simulink model "abs_SLX_CS9"  (R2020a)
settings: Solver=ode45  StartTime=0  StopTime=10  FixedStep=0.001  RelTol=1e-3  AbsTol=1e-6
libraries: Solver_SF x1
settings Model: ExtModeTrigMode=oneshot  ExtModeArmWhenConnect=off  Creator=jhu  LastModifiedBy=S288668
settings SolverCC: AutoScaleAbsTol=off
settings DataIOCC: SaveFormat=Array  SignalLoggingSaveFormat=ModelDataLogs  ReturnWorkspaceOutputs=off  SignalLoggingName=sigsOut
settings OptimizationCC: BlockReduction=off  BooleanDataType=off  ExpressionDepthLimit=2147483647  LifeSpan=inf
settings DebuggingCC: SaveWithParameterizedLinksMsg=none  UnderspecifiedInitializationDetection=Classic  MergeDetectMultiDrivingBlocksExec=none  SignalResolutionControl=TryResolveAllWithWarning  MultiTaskDSMMsg=warning  MultiTaskCondExecSysMsg=none  FcnCallInpInsideContextMsg=warning  StateNameClashWarn=warning  SFUnexpectedBacktrackingDiag=warning  SFNoUnconditionalDefaultTransitionDiag=warning  SFExecutionAtInitializationDiag=none  ArithmeticOperatorsInVariantConditions=warning
settings HardwareCC: ProdBitPerPointer=32  ProdBitPerSizeT=32  ProdBitPerPtrDiffT=32  ProdLargestAtomicFloat=None  ProdIntDivRoundTo=Undefined  ProdEndianess=Unspecified  ProdWordSize=32  ProdHWDeviceType=32-bit Generic  TargetUnknown=on
settings ModelReferenceCC: PropagateSignalLabelsOutOfModel=off
settings SFSimCC: SimUseLocalCustomCode=off  CustomCodeUndefinedFunction=UseInterfaceOnly
settings RTWCC: TemplateMakefile=grt_vc.tmf  RTWUseLocalCustomCode=off
settings CodeAppCC: StateflowObjectComments=on
settings GRTTargetCC: TargetFcnLib=ansi_tfl_tmw.mat  TargetLangStandard=C89/C90 (ANSI)  CombineOutputUpdateFcns=off  GRTInterface=on
settings ConfigComp: CovMetricSettings=dw  CovHtmlReporting=on  CovSaveCumulativeToWorkspaceVar=on  CovSaveSingleToWorkspaceVar=on  CovExternalEMLEnable=off

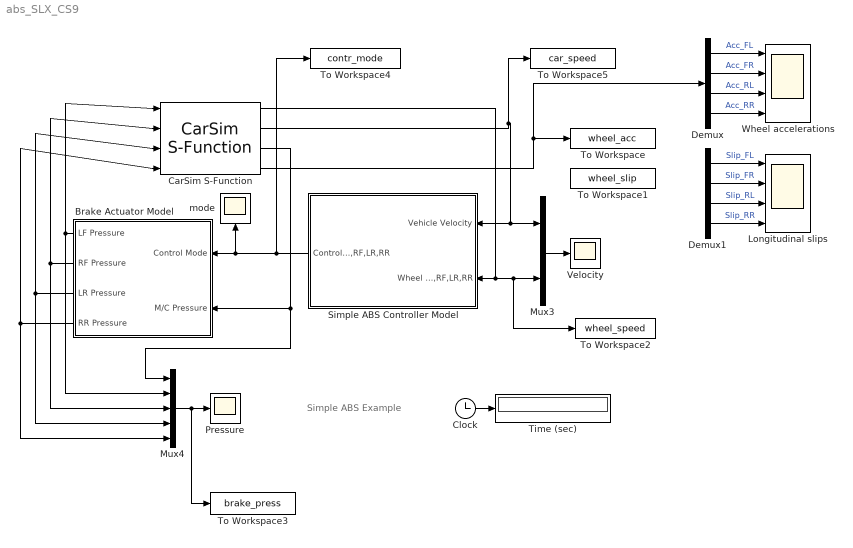
== system abs_SLX_CS9 ==
  note: Simple ABS Example
  Brake Actuator Model : Subsystem
  CarSim S-Function : Solver_SF/CarSim S-Function  Priority=1  SIMFILE=simfile.sim
  Clock : Clock
  Demux : Demux
  Demux1 : Demux
  Longitudinal slips : Scope  NumInputPorts=4
  Mux3 : Mux  Inputs=2
  Mux4 : Mux  Inputs=5
  Pressure : Scope
  Simple ABS Controller Model : Subsystem
  Time (sec) : Display
      settings: Format=bank  Decimation=100
  To Workspace : ToWorkspace  VariableName=wheel_acc  SaveFormat=Timeseries  SampleTime=-1
  To Workspace1 : ToWorkspace  VariableName=wheel_slip  SaveFormat=Timeseries  SampleTime=-1
  To Workspace2 : ToWorkspace  VariableName=wheel_speed  SaveFormat=Timeseries  SampleTime=-1
  To Workspace3 : ToWorkspace  VariableName=brake_press  SaveFormat=Timeseries  SampleTime=-1
  To Workspace4 : ToWorkspace  VariableName=contr_mode  SaveFormat=Timeseries  SampleTime=-1
  To Workspace5 : ToWorkspace  VariableName=car_speed  SaveFormat=Timeseries  SampleTime=-1
  Velocity : Scope
  Wheel accelerations : Scope  NumInputPorts=4
  mode : Scope
  wires:
  Mux4/1 -> To Workspace3/1, Pressure/1
  CarSim S-Function/2 -> To Workspace5/1, Mux3/1, Simple ABS Controller Model/1(Vehicle Velocity)
  CarSim S-Function/1 -> Simple ABS Controller Model/2(Wheel Velocity LF,RF,LR,RR), To Workspace2/1, Mux3/2
  Clock/1 -> Time (sec)/1
  Brake Actuator Model/1(LF Pressure) -> Mux4/2, CarSim S-Function/1
  Mux3/1 -> Velocity/1
  CarSim S-Function/3 -> Mux4/1, Brake Actuator Model/2(M/C Pressure)
  Brake Actuator Model/2(RF Pressure) -> Mux4/3, CarSim S-Function/2
  Brake Actuator Model/3(LR Pressure) -> Mux4/4, CarSim S-Function/3
  Brake Actuator Model/4(RR Pressure) -> Mux4/5, CarSim S-Function/4
  CarSim S-Function/4 -> Demux/1, To Workspace/1
  Demux/1 -> Wheel accelerations/1  "Acc_FL"
  Demux/2 -> Wheel accelerations/2  "Acc_FR"
  Demux/3 -> Wheel accelerations/3  "Acc_RL"
  Demux/4 -> Wheel accelerations/4  "Acc_RR"
  Demux1/4 -> Longitudinal slips/4  "Slip_RR"
  Demux1/3 -> Longitudinal slips/3  "Slip_RL"
  Demux1/2 -> Longitudinal slips/2  "Slip_FR"
  Demux1/1 -> Longitudinal slips/1  "Slip_FL"
  Simple ABS Controller Model/1(Control Mode LF,RF,LR,RR) -> mode/1, Brake Actuator Model/1(Control Mode), To Workspace4/1

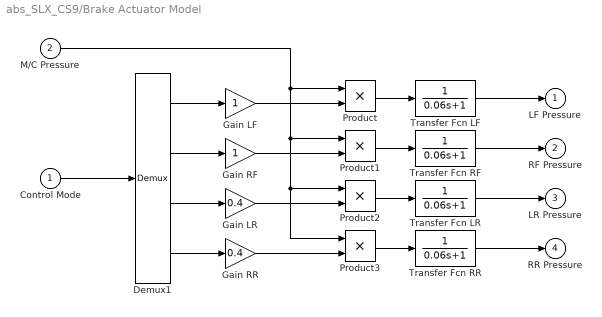
== system abs_SLX_CS9/Brake Actuator Model ==
  Control Mode : Inport
  M/C Pressure : Inport  Port=2
  Demux1 : Demux
      settings: DisplayOption=none
  Gain LF : Gain  SaturateOnIntegerOverflow=on  OutDataTypeStr=Inherit: Same as input  ParamDataTypeStr=Inherit: Same as input
  Gain LR : Gain  Gain=0.4  SaturateOnIntegerOverflow=on  OutDataTypeStr=Inherit: Same as input  ParamDataTypeStr=Inherit: Same as input
  Gain RF : Gain  SaturateOnIntegerOverflow=on  OutDataTypeStr=Inherit: Same as input  ParamDataTypeStr=Inherit: Same as input
  Gain RR : Gain  Gain=0.4  SaturateOnIntegerOverflow=on  OutDataTypeStr=Inherit: Same as input  ParamDataTypeStr=Inherit: Same as input
  Product{,1..3} (4 alike) : Product  InputSameDT=on  SaturateOnIntegerOverflow=on  OutDataTypeStr=Inherit: Same as first input
  Transfer Fcn LF : TransferFcn  Denominator=[0.06 1]
  Transfer Fcn LR : TransferFcn  Denominator=[0.06 1]
  Transfer Fcn RF : TransferFcn  Denominator=[0.06 1]
  Transfer Fcn RR : TransferFcn  Denominator=[0.06 1]
  LF Pressure : Outport  InitialOutput=0
  RF Pressure : Outport  Port=2  InitialOutput=0
  LR Pressure : Outport  Port=3  InitialOutput=0
  RR Pressure : Outport  Port=4  InitialOutput=0
  wires:
  Control Mode/1 -> Demux1/1
  Gain LF/1 -> Product/2
  Gain RF/1 -> Product1/2
  Gain LR/1 -> Product2/2
  Gain RR/1 -> Product3/2
  M/C Pressure/1 -> Product/1, Product1/1, Product2/1, Product3/1
  Product/1 -> Transfer Fcn LF/1
  Transfer Fcn LF/1 -> LF Pressure/1
  Product1/1 -> Transfer Fcn RF/1
  Product2/1 -> Transfer Fcn LR/1
  Product3/1 -> Transfer Fcn RR/1
  Transfer Fcn RF/1 -> RF Pressure/1
  Transfer Fcn LR/1 -> LR Pressure/1
  Transfer Fcn RR/1 -> RR Pressure/1
  Demux1/1 -> Gain LF/1
  Demux1/2 -> Gain RF/1
  Demux1/3 -> Gain LR/1
  Demux1/4 -> Gain RR/1

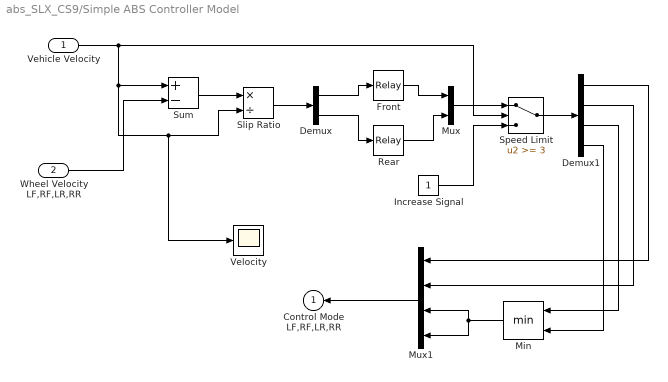
== system abs_SLX_CS9/Simple ABS Controller Model ==
  Vehicle Velocity : Inport
  Wheel Velocity LF,RF,LR,RR : Inport  Port=2
  Demux : Demux  Outputs=[2 2]
      settings: DisplayOption=none
  Demux1 : Demux
      settings: DisplayOption=none
  Front : Relay  OnSwitchValue=0.1  OffSwitchValue=0.05  OnOutputValue=0  OffOutputValue=1
  Increase Signal : Constant
  Min : MinMax  Inputs=2  InputSameDT=on  SaturateOnIntegerOverflow=on
  Mux : Mux  Inputs=2
  Mux1 : Mux
  Rear : Relay  OnSwitchValue=0.1  OffSwitchValue=0.05  OnOutputValue=0  OffOutputValue=1
  Slip Ratio : Product  Inputs=*/  InputSameDT=on  SaturateOnIntegerOverflow=on  OutDataTypeStr=Inherit: Same as first input
  Speed Limit : Switch  Threshold=3  SaturateOnIntegerOverflow=on  InputSameDT=on
  Sum : Sum  Inputs=+-  InputSameDT=on  SaturateOnIntegerOverflow=on  OutDataTypeStr=Inherit: Same as first input
  Velocity : Scope
  Control Mode LF,RF,LR,RR : Outport  InitialOutput=0
  wires:
  Vehicle Velocity/1 -> Sum/1, Slip Ratio/2, Velocity/1, Speed Limit/2
  Speed Limit/1 -> Demux1/1
  Increase Signal/1 -> Speed Limit/3
  Sum/1 -> Slip Ratio/1
  Slip Ratio/1 -> Demux/1
  Mux/1 -> Speed Limit/1
  Min/1 -> Mux1/3, Mux1/4
  Demux1/3 -> Min/1
  Demux1/4 -> Min/2
  Demux1/2 -> Mux1/2
  Demux1/1 -> Mux1/1
  Mux1/1 -> Control Mode LF,RF,LR,RR/1
  Front/1 -> Mux/1
  Demux/1 -> Front/1
  Demux/2 -> Rear/1
  Rear/1 -> Mux/2
  Wheel Velocity LF,RF,LR,RR/1 -> Sum/2
